simulink model "b"  (R2018a)
settings: Solver=VariableStepAuto  StartTime=0.0  StopTime=50.0  RelTol=1e-3
undefined symbols (not defined in the file): K_c, K_r
libraries: cstblocks x1, simulink x1
settings Model: Creator=Ale  LastModifiedBy=Ale

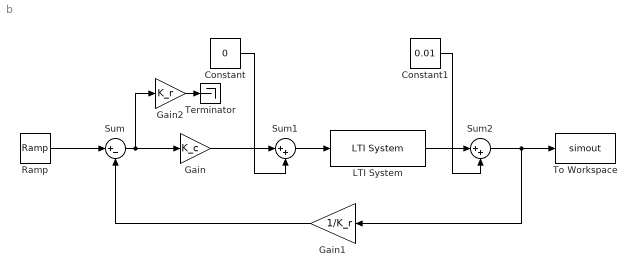
== system b ==
  Constant : Constant  Value=0
  Constant1 : Constant  Value=0.01
  Gain : Gain  Gain=K_c
  Gain1 : Gain  Gain=1/K_r
  Gain2 : Gain  Gain=K_r
  LTI System : cstblocks/LTI System  sys=F  IC=[]
  Ramp : simulink/Sources/Ramp  slope=2  start=0  InitialOutput=0
  Sum : Sum  Inputs=|+-
  Sum1 : Sum  Inputs=|++
  Sum2 : Sum  Inputs=|++
  Terminator : Terminator
  To Workspace : ToWorkspace  VariableName=simout  SaveFormat=Timeseries  SampleTime=-1
  wires:
  Gain2/1 -> Terminator/1
  Sum/1 -> Gain2/1, Gain/1
  Gain1/1 -> Sum/2
  Sum2/1 -> Gain1/1, To Workspace/1
  Constant1/1 -> Sum2/2
  LTI System/1 -> Sum2/1
  Sum1/1 -> LTI System/1
  Constant/1 -> Sum1/2
  Ramp/1 -> Sum/1
  Gain/1 -> Sum1/1
